simulink model "simulink_model"  (R2022b)
settings: Solver=VariableStepAuto  StartTime=0.0  StopTime=10.0  RelTol=1e-3
values from neighbouring files (symbols this model uses):
  A = [ 0                  ,1                     ,0                  ,0 ... (first row only)    [Inverted_pendulum_cart.m]
  B = [ 0 ... (first row only)    [Inverted_pendulum_cart.m]
settings Model: Creator=SIDDHARTH  LastModifiedBy=SIDDHARTH

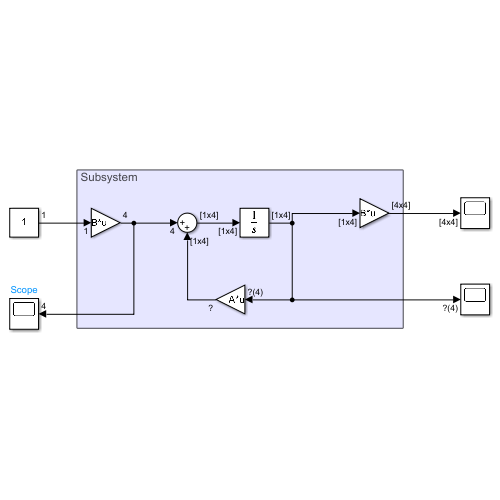
[thumbnail: Simulink's stored preview of the top-level diagram]
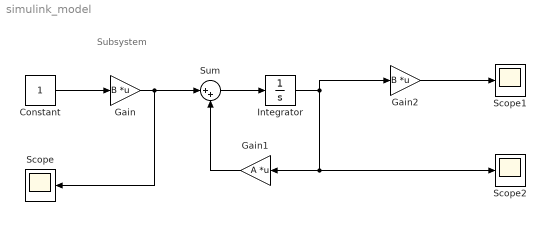
== system simulink_model ==
  note: Subsystem
  Constant : Constant
  Gain : Gain  Gain=B  Multiplication=Matrix(K*u)
  Gain1 : Gain  Gain=A  Multiplication=Matrix(K*u)
  Gain2 : Gain  Gain=B  Multiplication=Matrix(K*u)
  Integrator : Integrator
  Scope : Scope
  Scope1 : Scope
  Scope2 : Scope
  Sum : Sum  Inputs=|++
  wires:
  Integrator/1 -> Gain2/1, Scope2/1, Gain1/1
  Gain1/1 -> Sum/2
  Constant/1 -> Gain/1
  Sum/1 -> Integrator/1
  Gain/1 -> Scope/1, Sum/1
  Gain2/1 -> Scope1/1
